simulink model "Lab1_Part2"  (R2022b)
settings: Solver=VariableStepAuto  StartTime=0.0  StopTime=10.0  RelTol=1e-3
settings Model: Creator=Sahaj Singh  LastModifiedBy=Sahaj Singh

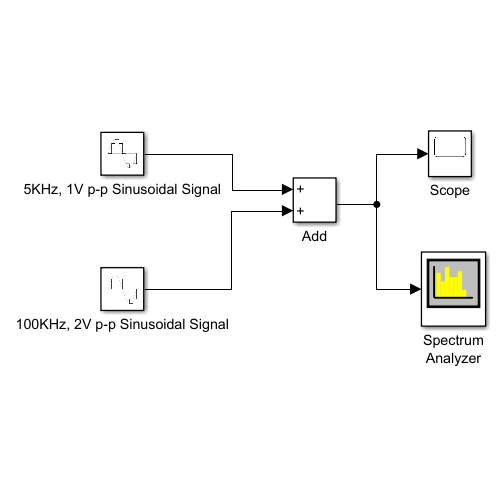
[thumbnail: Simulink's stored preview of the top-level diagram]
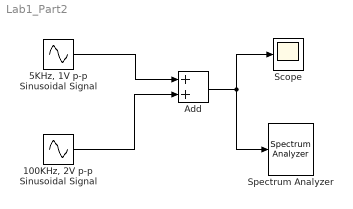
== system Lab1_Part2 ==
  "100KHz, 2V p-p Sinusoidal Signal" : Sin  Amplitude=2  Frequency=628318.53  SampleTime=1/100000
  "5KHz, 1V p-p Sinusoidal Signal" : Sin  Frequency=31415.9265  SampleTime=1/5000
  Add : Sum
  Scope : Scope
  Spectrum Analyzer : SpectrumAnalyzer
  wires:
  "5KHz, 1V p-p Sinusoidal Signal"/1 -> Add/1
  "100KHz, 2V p-p Sinusoidal Signal"/1 -> Add/2
  Add/1 -> Spectrum Analyzer/1, Scope/1
